simulink model "dc_motor_simulink"  (R2014b)
settings: Solver=ode45  StartTime=0.0  StopTime=1  RelTol=1e-3
values from neighbouring files (symbols this model uses):
  Bm = 0.01    [d_1_dc_motor_parameter.m]    (also in d_2_draw_wt_theta_real.m; d_2_draw_wt_theta_tf.m; d_4_dc_motor_bar_parameter.m; plot.m)
  Jm = 0.000052    (= 5.2e-05)    [d_1_dc_motor_parameter.m]    (also in d_2_draw_wt_theta_real.m; d_2_draw_wt_theta_tf.m; d_4_dc_motor_bar_parameter.m; plot.m)
  Ke = 0.235    [d_1_dc_motor_parameter.m]    (also in d_2_draw_wt_theta_real.m; d_2_draw_wt_theta_tf.m; d_4_dc_motor_bar_parameter.m; plot.m)
  Kt = 0.235    [d_1_dc_motor_parameter.m]    (also in d_2_draw_wt_theta_real.m; d_2_draw_wt_theta_tf.m; d_4_dc_motor_bar_parameter.m; plot.m)
  La = 0.23    [d_1_dc_motor_parameter.m]    (also in d_2_draw_wt_theta_real.m; d_2_draw_wt_theta_tf.m; d_4_dc_motor_bar_parameter.m; plot.m)
  Ra = 2    [d_1_dc_motor_parameter.m]    (also in d_2_draw_wt_theta_real.m; d_2_draw_wt_theta_tf.m; d_4_dc_motor_bar_parameter.m; plot.m)
settings Model: Creator=Admin  LastModifiedBy=Admin

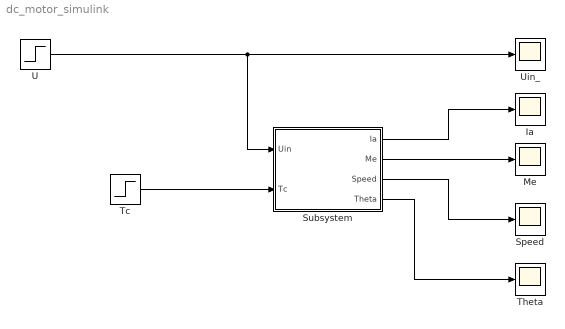
== system dc_motor_simulink ==
  Ia : Scope
      settings: YMin=0  YMax=10  SaveName=ScopeData2
  Me : Scope
      settings: YMin=0  YMax=10
  Speed : Scope
      settings: TimeRange=1.706369139607597  YMin=-34267.66  YMax=-34267.56000000001
  Subsystem : Subsystem
  Tc : Step  Time=0.5  After=0  SampleTime=0
  Theta : Scope
      settings: TimeRange=1.706369139607597  YMin=-34267.66  YMax=-34267.56000000001  SaveName=ScopeData4
  U : Step  Time=0.5  Before=12  After=-12  SampleTime=0
  Uin_ : Scope
      settings: TimeRange=1  YMin=0  YMax=10  SaveName=ScopeData3
  wires:
  Tc/1 -> Subsystem/2(Tc)
  Subsystem/1(Ia) -> Ia/1
  Subsystem/2(Me) -> Me/1
  Subsystem/3(Speed) -> Speed/1
  U/1 -> Subsystem/1(Uin), Uin_/1
  Subsystem/4(Theta) -> Theta/1

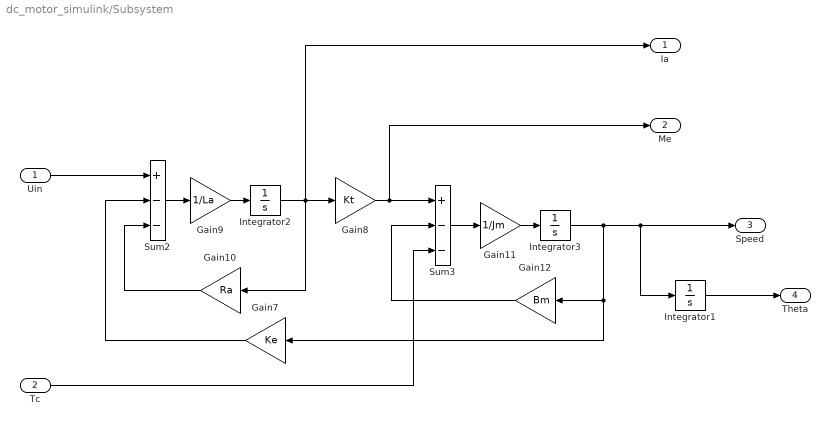
== system dc_motor_simulink/Subsystem ==
  Uin : Inport
  Tc : Inport  Port=2
  Gain10 : Gain  Gain=Ra
  Gain11 : Gain  Gain=1/Jm
  Gain12 : Gain  Gain=Bm
  Gain7 : Gain  Gain=Ke
  Gain8 : Gain  Gain=Kt
  Gain9 : Gain  Gain=1/La
  Integrator1 : Integrator
  Integrator2 : Integrator
  Integrator3 : Integrator
  Sum2 : Sum  Inputs=+--
  Sum3 : Sum  Inputs=+--
  Ia : Outport
  Me : Outport  Port=2
  Speed : Outport  Port=3
  Theta : Outport  Port=4
  wires:
  Gain7/1 -> Sum2/2
  Sum2/1 -> Gain9/1
  Gain10/1 -> Sum2/3
  Gain8/1 -> Me/1, Sum3/1
  Sum3/1 -> Gain11/1
  Gain9/1 -> Integrator2/1
  Gain12/1 -> Sum3/2
  Integrator3/1 -> Integrator1/1, Speed/1, Gain7/1, Gain12/1
  Integrator2/1 -> Ia/1, Gain10/1, Gain8/1
  Gain11/1 -> Integrator3/1
  Uin/1 -> Sum2/1
  Tc/1 -> Sum3/3
  Integrator1/1 -> Theta/1
